simulink model "Simulink_EbolaLineal"  (R2021b)
settings: Solver=VariableStepAuto  StartTime=0.0  StopTime=100.0  FixedStep=0.00126939799450362  RelTol=1e-3
model workspace (MAT data in the model file):
  Beta = 1.89e-07
  C = 8
  Delta = 0.0055
  P = 378
  U = 500
  Uu = 250
  V0 = 1.05
  u = 250
settings Model: Creator=Camilo  LastModifiedBy=Camilo
settings DataIOCC: SaveFormat=Array  OutputTimes=tout

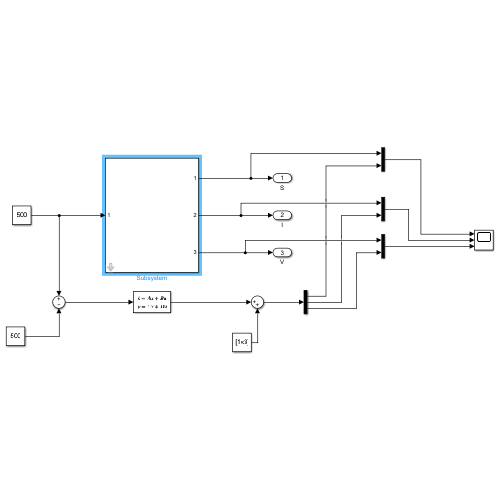
[thumbnail: Simulink's stored preview of the top-level diagram]
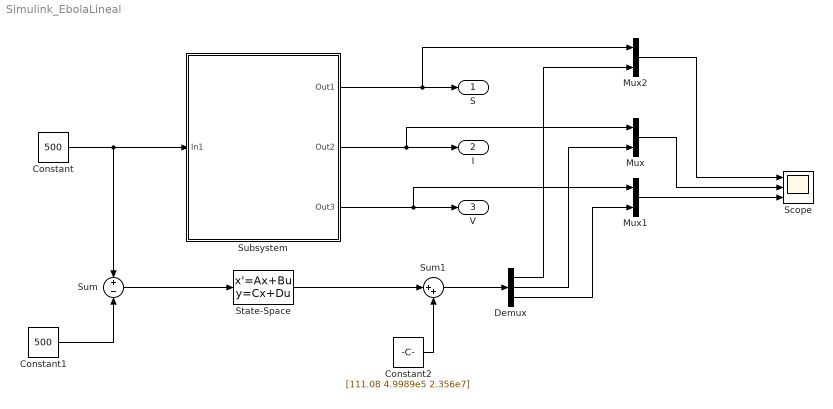
== system Simulink_EbolaLineal ==
  Constant : Constant  Value=500
  Constant1 : Constant  Value=500
  Constant2 : Constant  Value=[111.08 4.9989e5 2.356e7]
  Demux : Demux  Outputs=3
  Mux : Mux  Inputs=2
  Mux1 : Mux  Inputs=2
  Mux2 : Mux  Inputs=2
  Scope : Scope  NumInputPorts=3
  State-Space : StateSpace  A=|  B=[1 0 0]'  C=[1 0 0; 0 1 0; 0 0 1]  D=[0 0 0]'  InitialCondition=[0 0 0]
      | [-4.5010 0 0
      | ;4.5000 -0.0010 0.0000; 0 378.0000 -8.0200
      | 
      | ]
  Subsystem : Subsystem  mask{V0=2.3561e7, Delta=1e-3, P=378, C=8.02, Beta=1.91e-7}
  Sum : Sum  Inputs=+-
  Sum1 : Sum  Inputs=|++
  S : Outport
  I : Outport  Port=2
  V : Outport  Port=3
  wires:
  Subsystem/2(Out2) -> Mux/1, I/1
  Subsystem/3(Out3) -> V/1, Mux1/1
  Constant1/1 -> Sum/2
  Constant/1 -> Sum/1, Subsystem/1(In1)
  Sum/1 -> State-Space/1
  State-Space/1 -> Sum1/1
  Constant2/1 -> Sum1/2
  Sum1/1 -> Demux/1
  Subsystem/1(Out1) -> Mux2/1, S/1
  Demux/1 -> Mux2/2
  Demux/2 -> Mux/2
  Demux/3 -> Mux1/2
  Mux2/1 -> Scope/1
  Mux/1 -> Scope/2
  Mux1/1 -> Scope/3

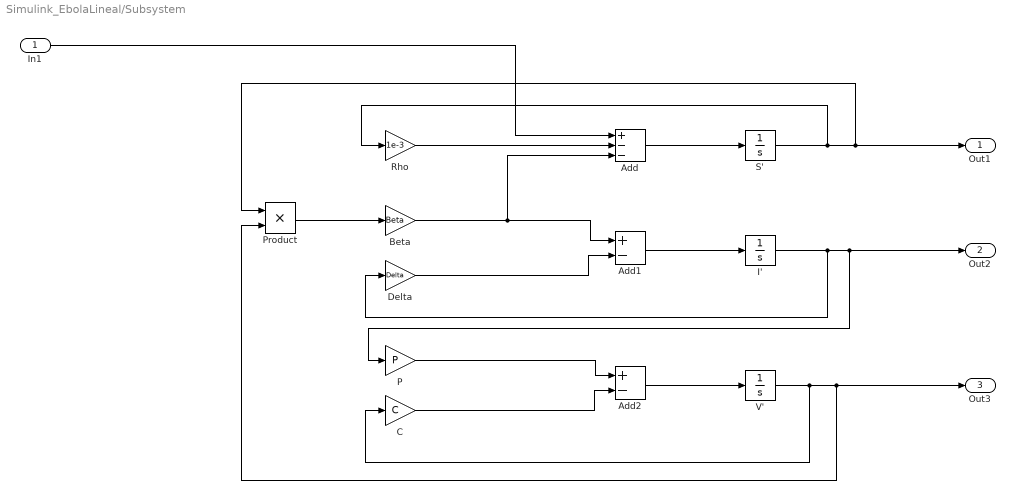
== system Simulink_EbolaLineal/Subsystem ==
  In1 : Inport
  Add : Sum  Inputs=+--
  Add1 : Sum  Inputs=+-
  Add2 : Sum  Inputs=+-
  Beta : Gain  Gain=Beta
  C : Gain  Gain=C
  Delta : Gain  Gain=Delta
  I' : Integrator  InitialCondition=4.9989e5  LimitOutput=on  LowerSaturationLimit=0
  P : Gain  Gain=P
  Product : Product
  Rho : Gain  Gain=1e-3
  S' : Integrator  InitialCondition=111.0834  LimitOutput=on  LowerSaturationLimit=0
  V' : Integrator  InitialCondition=V0  LimitOutput=on  LowerSaturationLimit=0
  Out1 : Outport
  Out2 : Outport  Port=2
  Out3 : Outport  Port=3
  wires:
  Add/1 -> S'/1
  C/1 -> Add2/2
  Beta/1 -> Add1/1, Add/3
  I'/1 -> Out2/1, P/1, Delta/1
  P/1 -> Add2/1
  S'/1 -> Out1/1, Product/1, Rho/1
  Rho/1 -> Add/2
  V'/1 -> Out3/1, Product/2, C/1
  Add2/1 -> V'/1
  Product/1 -> Beta/1
  Add1/1 -> I'/1
  Delta/1 -> Add1/2
  In1/1 -> Add/1
